simulink model "SF106A_MotRplCoggCfg"  (R2013b)
settings: Solver=FixedStepDiscrete  SolverMode=SingleTasking  StartTime=0.0  StopTime=1  FixedStep=0.002  RelTol=1e-3
undefined symbols (not defined in the file): ARCHGLBPRM_2PI_ULS_F32, ARCHGLBPRM_FLOATZEROTHD_ULS_F32, ARCHGLBPRM_HALFSQRT3_ULS_F32, COGGORDER1_CNT_U16, COGGORDER2_CNT_U16, COGGORDER3_CNT_U16, magnitude, MotCtrlPrmEstimnMotBackEmfConNom, MotRplCoggCfgMotAgTiDly, MotRplCoggCfgMotCurrDaxRplBilnrSeln, MotRplCoggCfgMotCurrQaxRpl, MotRplCoggCfgMotTqRplOrder1X, MotRplCoggCfgMotTqRplOrder1Y, MotRplCoggCfgMotTqRplOrder2X, MotRplCoggCfgMotTqRplOrder2Y, MotRplCoggCfgMotTqRplOrder3X, MotRplCoggCfgMotTqRplOrder3Y, MotRplCoggCmdHrmncOrder1Elec, MotRplCoggCmdHrmncOrder2Elec, MotRplCoggCmdHrmncOrder3Elec, NvmGetErrSts1, ONEOVER2_ULS_F32, SysGlbPrmMotPoleCnt, THREEOVER8_ULS_F32
libraries: NxtrLim x20, FixdToFloat x12, FloatToFixd x6, BilnrIntrpnCmnX x6, BilnrIntrpnCmnXDyn x6, NxtrMath x6, NxtrAbslt x5, NxtrNvM x3, simulink x2, NxtrSign x2
(part 2 of 3)

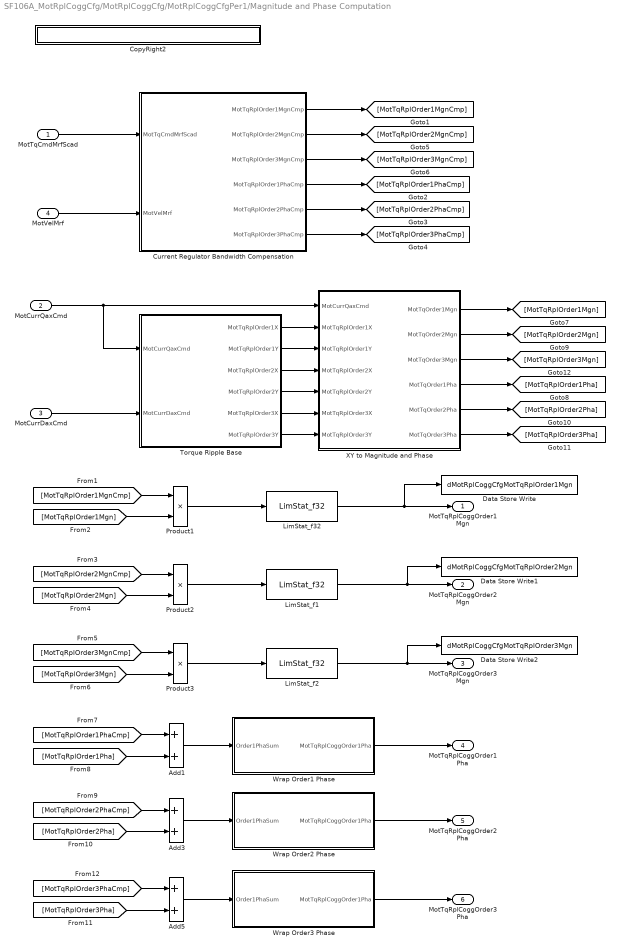
== system SF106A_MotRplCoggCfg/MotRplCoggCfg/MotRplCoggCfgPer1/Magnitude and Phase Computation ==
  MotTqCmdMrfScad : Inport
  MotCurrQaxCmd : Inport  Port=2
  MotCurrDaxCmd : Inport  Port=3
  MotVelMrf : Inport  Port=4
  Add1 : Sum  RequirementInfo="{'linktype_rmi_doors' '0000bb45 (/E-STEER Core/SubSystem Specifications/Application Functions/SF99/SF106A Cogging and Ripple Configuration)' '#SF106A_71' 'true' 'REQ:  SF106A_71' '' } %GIDa_648c56d2_593f_4874_8e89_241910faf26d"
  Add3 : Sum  RequirementInfo="{'linktype_rmi_doors' '0000bb45 (/E-STEER Core/SubSystem Specifications/Application Functions/SF99/SF106A Cogging and Ripple Configuration)' '#SF106A_71' 'true' 'REQ:  SF106A_71' '' } %GIDa_9a9eb539_2504_450c_99aa_20a14d3eef33"
  Add5 : Sum  RequirementInfo="{'linktype_rmi_doors' '0000bb45 (/E-STEER Core/SubSystem Specifications/Application Functions/SF99/SF106A Cogging and Ripple Configuration)' '#SF106A_71' 'true' 'REQ:  SF106A_71' '' } %GIDa_c4a088ef_46a4_443e_8376_4120059d3c17"
  CopyRight2 : Subsystem  Description=|  mask(Copyright Information){none=on}
      | Copyright info block.                                               
      |                                                                     
      | Place copyright information at the top of every subsystem in design.
      mask prompts: none "No parameters"
      mask help: Place copyright information at the top of every subsystem in design.
      mask Display:
      | NxtrConf = 'Nexteer Confidential';
      | 
      | sys = bdroot; %handle for the current model ("system")
      | first = get_param(sys,'Created');
      | if(isempty(first))
      |     first = datestr(now,'yyyy');
      | else
      |     first = first(end-3:end);  %year is last four digits
      | end
      | 
      | last = get_param(sys,'LastModifiedDate');
      | if isempty(last)
      |     last = datestr(now,'yyyy');
      | else
      |     last = last(end-3:end);
      | end
      | 
      | if strcmp(first,last)
      |     fprintf('%s -- Copyright %s Nexteer',NxtrConf,first)
      | else
      |     fprintf('%s -- %s%s- %s Nexteer',NxtrConf,char(169),first,last)
      | end
  Current Regulator Bandwidth Compensation : Subsystem
  Data Store Write : DataStoreWrite  DataStoreName=dMotRplCoggCfgMotTqRplOrder1Mgn
  Data Store Write1 : DataStoreWrite  DataStoreName=dMotRplCoggCfgMotTqRplOrder2Mgn
  Data Store Write2 : DataStoreWrite  DataStoreName=dMotRplCoggCfgMotTqRplOrder3Mgn
  LimStat_f1 : NxtrLim/LimStat_f32  RequirementInfo="{'linktype_rmi_doors' '0000bb45 (/E-STEER Core/SubSystem Specifications/Application Functions/SF99/SF106A Cogging and Ripple Configuration)' '#SF106A_65' 'true' 'REQ:  SF106A_65' '' } %GIDa_ccff9e31_03fc_44e9_a83d_9653ae9d67c5"  LoLim=MOTTQRPLLOLIM_MOTNWTMTR_F32  HiLim=MOTTQRPLHILIM_MOTNWTMTR_F32
      settings: AttributesFormatString=|
      | Low Limit: %<LoLim>
      | High Limit:%<HiLim>
  LimStat_f2 : NxtrLim/LimStat_f32  RequirementInfo="{'linktype_rmi_doors' '0000bb45 (/E-STEER Core/SubSystem Specifications/Application Functions/SF99/SF106A Cogging and Ripple Configuration)' '#SF106A_65' 'true' 'REQ:  SF106A_65' '' } %GIDa_ae5aa3cb_1ae4_4be4_adae_075219de67e5"  LoLim=MOTTQRPLLOLIM_MOTNWTMTR_F32  HiLim=MOTTQRPLHILIM_MOTNWTMTR_F32
      settings: AttributesFormatString=|
      | Low Limit: %<LoLim>
      | High Limit:%<HiLim>
  LimStat_f32 : NxtrLim/LimStat_f32  RequirementInfo="{'linktype_rmi_doors' '0000bb45 (/E-STEER Core/SubSystem Specifications/Application Functions/SF99/SF106A Cogging and Ripple Configuration)' '#SF106A_65' 'true' 'REQ:  SF106A_65' '' } %GIDa_ba4c2155_2466_4bb3_b693_debdd3d2d6c5"  LoLim=MOTTQRPLLOLIM_MOTNWTMTR_F32  HiLim=MOTTQRPLHILIM_MOTNWTMTR_F32
      settings: AttributesFormatString=|
      | Low Limit: %<LoLim>
      | High Limit:%<HiLim>
  Product1 : Product  RequirementInfo="{'linktype_rmi_doors' '0000bb45 (/E-STEER Core/SubSystem Specifications/Application Functions/SF99/SF106A Cogging and Ripple Configuration)' '#SF106A_70' 'true' 'REQ:  SF106A_70' '' } %GIDa_7ac384b6_01f3_4e7b_b1d7_d1b5b6b1e867"
  Product2 : Product  RequirementInfo="{'linktype_rmi_doors' '0000bb45 (/E-STEER Core/SubSystem Specifications/Application Functions/SF99/SF106A Cogging and Ripple Configuration)' '#SF106A_70' 'true' 'REQ:  SF106A_70' '' } %GIDa_9c353b42_6df7_4475_b5bc_a373fdcf9e44"
  Product3 : Product  RequirementInfo="{'linktype_rmi_doors' '0000bb45 (/E-STEER Core/SubSystem Specifications/Application Functions/SF99/SF106A Cogging and Ripple Configuration)' '#SF106A_70' 'true' 'REQ:  SF106A_70' '' } %GIDa_458a2e09_2cf4_40dd_a1d9_b337fe68f59e"
  Torque Ripple Base : Subsystem
  Wrap Order1 Phase : Subsystem  RequirementInfo="{'linktype_rmi_doors' '0000bb45 (/E-STEER Core/SubSystem Specifications/Application Functions/SF99/SF106A Cogging and Ripple Configuration)' '#SF106A_72' 'true' 'REQ:  SF106A_72' '' } %GIDa_d597ade6_de24_47ef_a527_55bbe8aaa597"
  Wrap Order2 Phase : Subsystem  RequirementInfo="{'linktype_rmi_doors' '0000bb45 (/E-STEER Core/SubSystem Specifications/Application Functions/SF99/SF106A Cogging and Ripple Configuration)' '#SF106A_72' 'true' 'REQ:  SF106A_72' '' } %GIDa_7d28c792_5d3e_45ce_b917_447f54703099"
  Wrap Order3 Phase : Subsystem  RequirementInfo="{'linktype_rmi_doors' '0000bb45 (/E-STEER Core/SubSystem Specifications/Application Functions/SF99/SF106A Cogging and Ripple Configuration)' '#SF106A_72' 'true' 'REQ:  SF106A_72' '' } %GIDa_e3528b43_aef0_489e_91c9_b2e9623abd20"
  XY to Magnitude and Phase : Subsystem
  MotTqRplCoggOrder1Mgn : Outport
  MotTqRplCoggOrder2Mgn : Outport  Port=2
  MotTqRplCoggOrder3Mgn : Outport  Port=3
  MotTqRplCoggOrder1Pha : Outport  Port=4
  MotTqRplCoggOrder2Pha : Outport  Port=5
  MotTqRplCoggOrder3Pha : Outport  Port=6
  wires:
  MotTqCmdMrfScad/1 -> Current Regulator Bandwidth Compensation/1(MotTqCmdMrfScad)
  MotCurrDaxCmd/1 -> Torque Ripple Base/2(MotCurrDaxCmd)
  Torque Ripple Base/6(MotTqRplOrder3Y) -> XY to Magnitude and Phase/7(MotTqRplOrder3Y)
  Torque Ripple Base/5(MotTqRplOrder3X) -> XY to Magnitude and Phase/6(MotTqRplOrder3X)
  Torque Ripple Base/1(MotTqRplOrder1X) -> XY to Magnitude and Phase/2(MotTqRplOrder1X)
  Torque Ripple Base/4(MotTqRplOrder2Y) -> XY to Magnitude and Phase/5(MotTqRplOrder2Y)
  Torque Ripple Base/2(MotTqRplOrder1Y) -> XY to Magnitude and Phase/3(MotTqRplOrder1Y)
  Torque Ripple Base/3(MotTqRplOrder2X) -> XY to Magnitude and Phase/4(MotTqRplOrder2X)
  MotCurrQaxCmd/1 -> XY to Magnitude and Phase/1(MotCurrQaxCmd), Torque Ripple Base/1(MotCurrQaxCmd)
  LimStat_f2/1 -> Data Store Write2/1, MotTqRplCoggOrder3Mgn/1
  LimStat_f1/1 -> MotTqRplCoggOrder2Mgn/1, Data Store Write1/1
  LimStat_f32/1 -> MotTqRplCoggOrder1Mgn/1, Data Store Write/1
  MotVelMrf/1 -> Current Regulator Bandwidth Compensation/2(MotVelMrf)
  Product1/1 -> LimStat_f32/1
  [MotTqRplOrder1MgnCmp] -> Product1/1
  [MotTqRplOrder1Mgn] -> Product1/2
  Product2/1 -> LimStat_f1/1
  [MotTqRplOrder2MgnCmp] -> Product2/1
  [MotTqRplOrder2Mgn] -> Product2/2
  Product3/1 -> LimStat_f2/1
  [MotTqRplOrder3MgnCmp] -> Product3/1
  [MotTqRplOrder3Mgn] -> Product3/2
  [MotTqRplOrder1Pha] -> Add1/2
  [MotTqRplOrder1PhaCmp] -> Add1/1
  [MotTqRplOrder2Pha] -> Add3/2
  [MotTqRplOrder2PhaCmp] -> Add3/1
  [MotTqRplOrder3Pha] -> Add5/2
  [MotTqRplOrder3PhaCmp] -> Add5/1
  Add1/1 -> Wrap Order1 Phase/1(Order1PhaSum)
  Wrap Order1 Phase/1(MotTqRplCoggOrder1Pha) -> MotTqRplCoggOrder1Pha/1
  Add3/1 -> Wrap Order2 Phase/1(Order1PhaSum)
  Wrap Order2 Phase/1(MotTqRplCoggOrder1Pha) -> MotTqRplCoggOrder2Pha/1
  Add5/1 -> Wrap Order3 Phase/1(Order1PhaSum)
  Wrap Order3 Phase/1(MotTqRplCoggOrder1Pha) -> MotTqRplCoggOrder3Pha/1
  XY to Magnitude and Phase/1(MotTqOrder1Mgn) -> [MotTqRplOrder1Mgn]
  XY to Magnitude and Phase/3(MotTqOrder3Mgn) -> [MotTqRplOrder3Mgn]
  XY to Magnitude and Phase/5(MotTqOrder2Pha) -> [MotTqRplOrder2Pha]
  XY to Magnitude and Phase/2(MotTqOrder2Mgn) -> [MotTqRplOrder2Mgn]
  XY to Magnitude and Phase/6(MotTqOrder3Pha) -> [MotTqRplOrder3Pha]
  XY to Magnitude and Phase/4(MotTqOrder1Pha) -> [MotTqRplOrder1Pha]
  Current Regulator Bandwidth Compensation/4(MotTqRplOrder1PhaCmp) -> [MotTqRplOrder1PhaCmp]
  Current Regulator Bandwidth Compensation/2(MotTqRplOrder2MgnCmp) -> [MotTqRplOrder2MgnCmp]
  Current Regulator Bandwidth Compensation/3(MotTqRplOrder3MgnCmp) -> [MotTqRplOrder3MgnCmp]
  Current Regulator Bandwidth Compensation/6(MotTqRplOrder3PhaCmp) -> [MotTqRplOrder3PhaCmp]
  Current Regulator Bandwidth Compensation/1(MotTqRplOrder1MgnCmp) -> [MotTqRplOrder1MgnCmp]
  Current Regulator Bandwidth Compensation/5(MotTqRplOrder2PhaCmp) -> [MotTqRplOrder2PhaCmp]

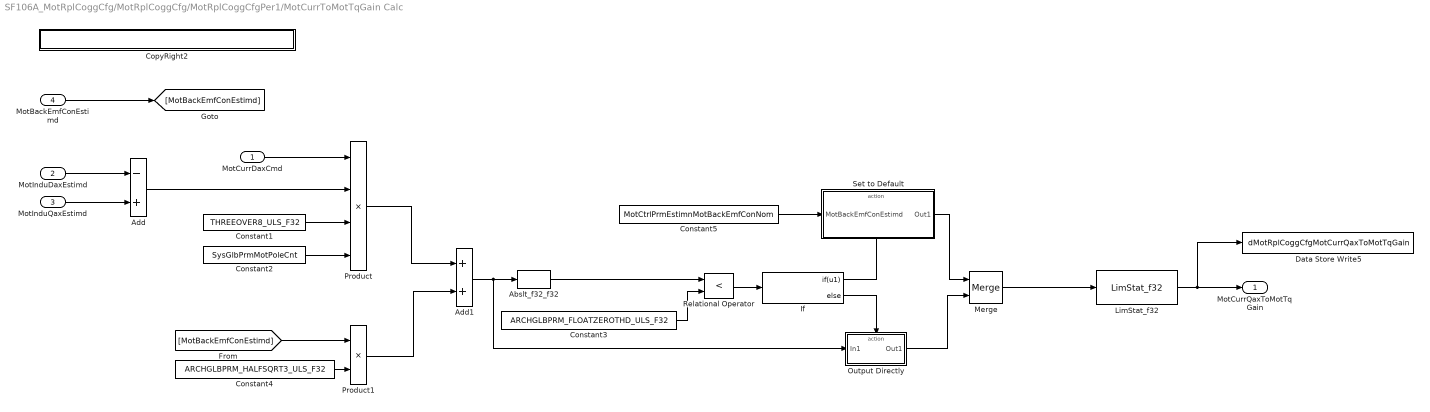
== system SF106A_MotRplCoggCfg/MotRplCoggCfg/MotRplCoggCfgPer1/MotCurrToMotTqGain Calc ==
  MotCurrDaxCmd : Inport
  MotInduDaxEstimd : Inport  Port=2
  MotInduQaxEstimd : Inport  Port=3
  MotBackEmfConEstimd : Inport  Port=4
  Abslt_f32_f32 : NxtrAbslt/Abslt_f32_f32  RequirementInfo="{'linktype_rmi_doors' '0000bb45 (/E-STEER Core/SubSystem Specifications/Application Functions/SF99/SF106A Cogging and Ripple Configuration)' '#SF106A_56' 'true' 'REQ:  SF106A_56' '' } %GIDa_3dd04d32_cbb3_4f3b_a584_375cf79a7190"  SFunctionSpec=single y1 = Abslt_f32_f32(single u1)
      settings: AttributesFormatString=%<Name>
  Add : Sum  RequirementInfo="{'linktype_rmi_doors' '0000bb45 (/E-STEER Core/SubSystem Specifications/Application Functions/SF99/SF106A Cogging and Ripple Configuration)' '#SF106A_54' 'true' 'REQ:  SF106A_54' '' } %GIDa_ba1b20c0_2ede_4be5_979a_b04b55223ef1"  Inputs=-+
  Add1 : Sum  RequirementInfo="{'linktype_rmi_doors' '0000bb45 (/E-STEER Core/SubSystem Specifications/Application Functions/SF99/SF106A Cogging and Ripple Configuration)' '#SF106A_54' 'true' 'REQ:  SF106A_54' '' } %GIDa_ee9a033f_945c_4511_8002_119d863c4908"
  Constant1 : Constant  Value=THREEOVER8_ULS_F32
  Constant2 : Constant  Value=SysGlbPrmMotPoleCnt
  Constant3 : Constant  Value=ARCHGLBPRM_FLOATZEROTHD_ULS_F32
  Constant4 : Constant  Value=ARCHGLBPRM_HALFSQRT3_ULS_F32
  Constant5 : Constant  RequirementInfo={'linktype_rmi_doors' '0000bb45 (/E-STEER Core/SubSystem Specifications/Application Functions/SF99/SF106A Cogging and Ripple Configuration)' '#SF106A_115' 'true' 'REQ: SF106A_115' '' } %GIDa_32d27978_b4ee_4bc2_b947_2a7fafd2bf6c  Value=MotCtrlPrmEstimnMotBackEmfConNom
  CopyRight2 : Subsystem  Description=|  mask(Copyright Information){none=on}
      | Copyright info block.                                               
      |                                                                     
      | Place copyright information at the top of every subsystem in design.
      mask prompts: none "No parameters"
      mask help: Place copyright information at the top of every subsystem in design.
      mask Display:
      | NxtrConf = 'Nexteer Confidential';
      | 
      | sys = bdroot; %handle for the current model ("system")
      | first = get_param(sys,'Created');
      | if(isempty(first))
      |     first = datestr(now,'yyyy');
      | else
      |     first = first(end-3:end);  %year is last four digits
      | end
      | 
      | last = get_param(sys,'LastModifiedDate');
      | if isempty(last)
      |     last = datestr(now,'yyyy');
      | else
      |     last = last(end-3:end);
      | end
      | 
      | if strcmp(first,last)
      |     fprintf('%s -- Copyright %s Nexteer',NxtrConf,first)
      | else
      |     fprintf('%s -- %s%s- %s Nexteer',NxtrConf,char(169),first,last)
      | end
  Data Store Write5 : DataStoreWrite  DataStoreName=dMotRplCoggCfgMotCurrQaxToMotTqGain
  If : If  RequirementInfo="{'linktype_rmi_doors' '0000bb45 (/E-STEER Core/SubSystem Specifications/Application Functions/SF99/SF106A Cogging and Ripple Configuration)' '#SF106A_56' 'true' 'REQ:  SF106A_56' '' ; 'linktype_rmi_doors' '0000bb45 (/E-STEER Core/SubSystem Specifications/Application Functions/SF99/SF106A Cogging and Ripple Configuration)' '#SF106A_56' 'true' 'REQ:  SF106A_56' '' } %GIDa_a5d88a30_9910_4f5f_9fc9_b7b9a6575954"  IfExpression=u1
  LimStat_f32 : NxtrLim/LimStat_f32  LoLim=MOTCURRQAXTOMOTTQGAINLOLIM_VOLTPERMOTRADPERSEC_F32  HiLim=MOTCURRQAXTOMOTTQGAINHILIM_VOLTPERMOTRADPERSEC_F32
      settings: AttributesFormatString=|
      | Low Limit: %<LoLim>
      | High Limit:%<HiLim>
  Merge : Merge  RequirementInfo="{'linktype_rmi_doors' '0000bb45 (/E-STEER Core/SubSystem Specifications/Application Functions/SF99/SF106A Cogging and Ripple Configuration)' '#SF106A_56' 'true' 'REQ:  SF106A_56' '' } %GIDa_c0409470_3f74_4a50_ab79_400dfe325cdd"
  Output Directly : Subsystem  RequirementInfo="{'linktype_rmi_doors' '0000bb45 (/E-STEER Core/SubSystem Specifications/Application Functions/SF99/SF106A Cogging and Ripple Configuration)' '#SF106A_56' 'true' 'REQ:  SF106A_56' '' } %GIDa_2b70c7c7_a78b_446c_bf60_f39fcd5329cf"  TreatAsAtomicUnit=on
  Product : Product  RequirementInfo="{'linktype_rmi_doors' '0000bb45 (/E-STEER Core/SubSystem Specifications/Application Functions/SF99/SF106A Cogging and Ripple Configuration)' '#SF106A_54' 'true' 'REQ:  SF106A_54' '' } %GIDa_d7691117_ecce_48e1_9f0c_630d5d46c3ee"  Inputs=4
  Product1 : Product  RequirementInfo="{'linktype_rmi_doors' '0000bb45 (/E-STEER Core/SubSystem Specifications/Application Functions/SF99/SF106A Cogging and Ripple Configuration)' '#SF106A_54' 'true' 'REQ:  SF106A_54' '' } %GIDa_d73ba26f_a7f2_4740_a78f_0423572b7171"
  Relational Operator : RelationalOperator  RequirementInfo="{'linktype_rmi_doors' '0000bb45 (/E-STEER Core/SubSystem Specifications/Application Functions/SF99/SF106A Cogging and Ripple Configuration)' '#SF106A_56' 'true' 'REQ:  SF106A_56' '' } %GIDa_6b39b974_a2b5_4090_81ce_b211ed84d319"  Operator=<  OutDataTypeStr=boolean
  Set to Default : Subsystem  RequirementInfo="{'linktype_rmi_doors' '0000bb45 (/E-STEER Core/SubSystem Specifications/Application Functions/SF99/SF106A Cogging and Ripple Configuration)' '#SF106A_56' 'true' 'REQ:  SF106A_56' '' } %GIDa_e7fae6b2_5e55_4c14_bb87_5e4affbd739c"  TreatAsAtomicUnit=on
  MotCurrQaxToMotTqGain : Outport
  wires:
  MotInduQaxEstimd/1 -> Add/2
  MotInduDaxEstimd/1 -> Add/1
  Add/1 -> Product/2
  Constant2/1 -> Product/4
  Constant1/1 -> Product/3
  Constant4/1 -> Product1/2
  MotBackEmfConEstimd/1 -> [MotBackEmfConEstimd]
  MotCurrDaxCmd/1 -> Product/1
  Product/1 -> Add1/1
  Product1/1 -> Add1/2
  Add1/1 -> Output Directly/1(In1), Abslt_f32_f32/1
  If/2 -> Output Directly/Action
  If/1 -> Set to Default/Action
  Set to Default/1(Out1) -> Merge/1
  Output Directly/1(Out1) -> Merge/2
  [MotBackEmfConEstimd] -> Product1/1
  Merge/1 -> LimStat_f32/1
  Abslt_f32_f32/1 -> Relational Operator/1
  LimStat_f32/1 -> Data Store Write5/1, MotCurrQaxToMotTqGain/1
  Relational Operator/1 -> If/1
  Constant3/1 -> Relational Operator/2
  Constant5/1 -> Set to Default/1(MotBackEmfConEstimd)

== system SF106A_MotRplCoggCfg/MotRplCoggCfg/MotRplCoggCfgPer1/Position Delay ==
  MotVelMrf : Inport
  Constant : Constant  Value=SysGlbPrmMotPoleCnt
  Constant1 : Constant  Value=ONEOVER2_ULS_F32
  Constant2 : Constant  Value=MotRplCoggCfgMotAgTiDly
  CopyRight2 : Subsystem  Description=|  mask(Copyright Information){none=on}
      | Copyright info block.                                               
      |                                                                     
      | Place copyright information at the top of every subsystem in design.
      mask prompts: none "No parameters"
      mask help: Place copyright information at the top of every subsystem in design.
      mask Display:
      | NxtrConf = 'Nexteer Confidential';
      | 
      | sys = bdroot; %handle for the current model ("system")
      | first = get_param(sys,'Created');
      | if(isempty(first))
      |     first = datestr(now,'yyyy');
      | else
      |     first = first(end-3:end);  %year is last four digits
      | end
      | 
      | last = get_param(sys,'LastModifiedDate');
      | if isempty(last)
      |     last = datestr(now,'yyyy');
      | else
      |     last = last(end-3:end);
      | end
      | 
      | if strcmp(first,last)
      |     fprintf('%s -- Copyright %s Nexteer',NxtrConf,first)
      | else
      |     fprintf('%s -- %s%s- %s Nexteer',NxtrConf,char(169),first,last)
      | end
  Data Store Write5 : DataStoreWrite  DataStoreName=dMotRplCoggCfgMotAgElecDlyRpl
  LimStat_f32 : NxtrLim/LimStat_f32  LoLim=MOTAGELECDLYRPLLOLIM_MOTRAD_F32  HiLim=MOTAGELECDLYRPLHILIM_MOTRAD_F32
      settings: AttributesFormatString=|
      | Low Limit: %<LoLim>
      | High Limit:%<HiLim>
  Product : Product  RequirementInfo="{'linktype_rmi_doors' '0000bb45 (/E-STEER Core/SubSystem Specifications/Application Functions/SF99/SF106A Cogging and Ripple Configuration)' '#SF106A_79' 'true' 'REQ:  SF106A_79' '' } %GIDa_afe57c97_f375_490a_8df4_4de7a5eb3ebb"  Inputs=4
  MotAgElecDlyRpl : Outport
  wires:
  MotVelMrf/1 -> Product/1
  Constant2/1 -> Product/2
  Constant/1 -> Product/3
  Constant1/1 -> Product/4
  Product/1 -> LimStat_f32/1
  LimStat_f32/1 -> Data Store Write5/1, MotAgElecDlyRpl/1

== system SF106A_MotRplCoggCfg/MotRplCoggCfg/SetMotRplCoggPrm/CopyRight2 ==

== system SF106A_MotRplCoggCfg/MotRplCoggCfg/MotRplCoggCfgInit1/NVM is NOT okay/CopyRight2 ==

== system SF106A_MotRplCoggCfg/MotRplCoggCfg/MotRplCoggCfgInit1/NVM is okay/CopyRight2 ==

== system SF106A_MotRplCoggCfg/MotRplCoggCfg/MotRplCoggCfgPer1/Magnitude and Phase Computation/CopyRight2 ==

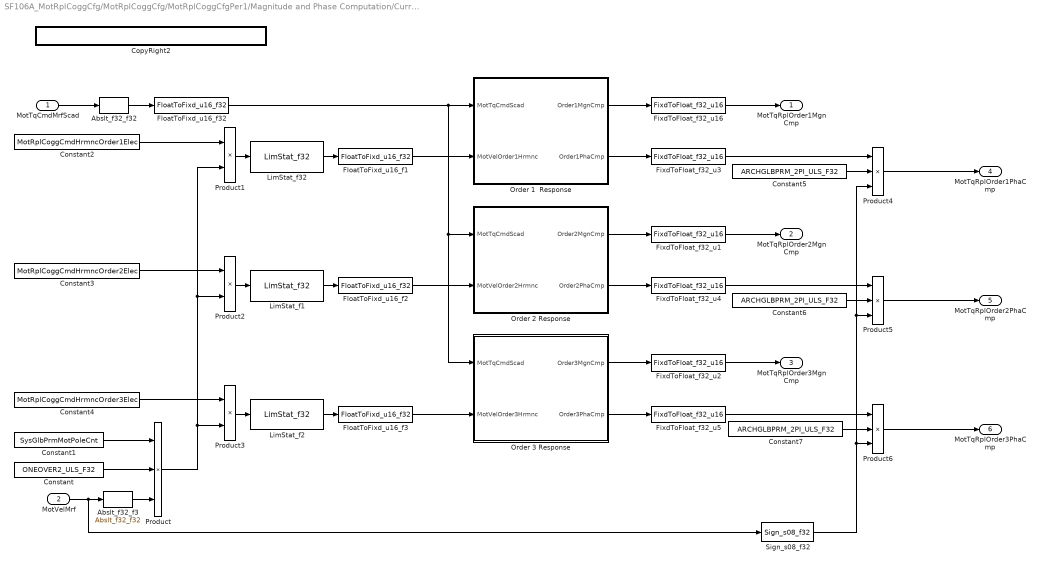
== system SF106A_MotRplCoggCfg/MotRplCoggCfg/MotRplCoggCfgPer1/Magnitude and Phase Computation/Current Regulator Bandwidth Compensation ==
  MotTqCmdMrfScad : Inport
  MotVelMrf : Inport  Port=2
  Abslt_f32_f3 : NxtrAbslt/Abslt_f32_f32  RequirementInfo="{'linktype_rmi_doors' '0000bb45 (/E-STEER Core/SubSystem Specifications/Application Functions/SF99/SF106A Cogging and Ripple Configuration)' '#SF106A_67' 'true' 'REQ:  SF106A_67' '' ; 'linktype_rmi_doors' '0000bb45 (/E-STEER Core/SubSystem Specifications/Application Functions/SF99/SF106A Cogging and Ripple Configuration)' '#SF106A_68' 'true' 'REQ:  SF106A_68' '' } %GIDa_33edf65c_2e46_411e_8167_82b34b9b363e"  SFunctionSpec=single y1 = Abslt_f32_f32(single u1)
      settings: AttributesFormatString=%<Name>
  Abslt_f32_f32 : NxtrAbslt/Abslt_f32_f32  RequirementInfo="{'linktype_rmi_doors' '0000bb45 (/E-STEER Core/SubSystem Specifications/Application Functions/SF99/SF106A Cogging and Ripple Configuration)' '#SF106A_67' 'true' 'REQ:  SF106A_67' '' ; 'linktype_rmi_doors' '0000bb45 (/E-STEER Core/SubSystem Specifications/Application Functions/SF99/SF106A Cogging and Ripple Configuration)' '#SF106A_68' 'true' 'REQ:  SF106A_68' '' } %GIDa_7d0e2c5c_7282_4961_ba80_71904d67d8ed"  SFunctionSpec=single y1 = Abslt_f32_f32(single u1)
      settings: AttributesFormatString=%<Name>
  Constant : Constant  Value=ONEOVER2_ULS_F32
  Constant1 : Constant  Value=SysGlbPrmMotPoleCnt
  Constant2 : Constant  Value=MotRplCoggCmdHrmncOrder1Elec
  Constant3 : Constant  Value=MotRplCoggCmdHrmncOrder2Elec
  Constant4 : Constant  Value=MotRplCoggCmdHrmncOrder3Elec
  Constant5 : Constant  Value=ARCHGLBPRM_2PI_ULS_F32
  Constant6 : Constant  Value=ARCHGLBPRM_2PI_ULS_F32
  Constant7 : Constant  Value=ARCHGLBPRM_2PI_ULS_F32
  CopyRight2 : Subsystem  Description=|  mask(Copyright Information){none=on}
      | Copyright info block.                                               
      |                                                                     
      | Place copyright information at the top of every subsystem in design.
      mask prompts: none "No parameters"
      mask help: Place copyright information at the top of every subsystem in design.
      mask Display:
      | NxtrConf = 'Nexteer Confidential';
      | 
      | sys = bdroot; %handle for the current model ("system")
      | first = get_param(sys,'Created');
      | if(isempty(first))
      |     first = datestr(now,'yyyy');
      | else
      |     first = first(end-3:end);  %year is last four digits
      | end
      | 
      | last = get_param(sys,'LastModifiedDate');
      | if isempty(last)
      |     last = datestr(now,'yyyy');
      | else
      |     last = last(end-3:end);
      | end
      | 
      | if strcmp(first,last)
      |     fprintf('%s -- Copyright %s Nexteer',NxtrConf,first)
      | else
      |     fprintf('%s -- %s%s- %s Nexteer',NxtrConf,char(169),first,last)
      | end
  FixdToFloat_f32_u1 : FixdToFloat/FixdToFloat_f32_u16  Param1=13
  FixdToFloat_f32_u16 : FixdToFloat/FixdToFloat_f32_u16  Param1=13
  FixdToFloat_f32_u2 : FixdToFloat/FixdToFloat_f32_u16  Param1=13
  FixdToFloat_f32_u3 : FixdToFloat/FixdToFloat_f32_u16  Param1=16
  FixdToFloat_f32_u4 : FixdToFloat/FixdToFloat_f32_u16  Param1=16
  FixdToFloat_f32_u5 : FixdToFloat/FixdToFloat_f32_u16  Param1=16
  FloatToFixd_u16_f1 : FloatToFixd/FloatToFixd_u16_f32  Param1=0
  FloatToFixd_u16_f2 : FloatToFixd/FloatToFixd_u16_f32  Param1=0
  FloatToFixd_u16_f3 : FloatToFixd/FloatToFixd_u16_f32  Param1=0
  FloatToFixd_u16_f32 : FloatToFixd/FloatToFixd_u16_f32  Param1=11
  LimStat_f1 : NxtrLim/LimStat_f32  LoLim=SCADMOTVELLOLIM_MOTRADPERSEC_F32  HiLim=SCADMOTVELHILIM_MOTRADPERSEC_F32
      settings: AttributesFormatString=|
      | Low Limit: %<LoLim>
      | High Limit:%<HiLim>
  LimStat_f2 : NxtrLim/LimStat_f32  LoLim=SCADMOTVELLOLIM_MOTRADPERSEC_F32  HiLim=SCADMOTVELHILIM_MOTRADPERSEC_F32
      settings: AttributesFormatString=|
      | Low Limit: %<LoLim>
      | High Limit:%<HiLim>
  LimStat_f32 : NxtrLim/LimStat_f32  LoLim=SCADMOTVELLOLIM_MOTRADPERSEC_F32  HiLim=SCADMOTVELHILIM_MOTRADPERSEC_F32
      settings: AttributesFormatString=|
      | Low Limit: %<LoLim>
      | High Limit:%<HiLim>
  Order 1  Response : Subsystem
  Order 2 Response : Subsystem
  Order 3 Response : Subsystem
  Product : Product  RequirementInfo="{'linktype_rmi_doors' '0000bb45 (/E-STEER Core/SubSystem Specifications/Application Functions/SF99/SF106A Cogging and Ripple Configuration)' '#SF106A_81' 'true' 'REQ:  SF106A_81' '' } %GIDa_c32ba144_8f46_4563_9287_d3fbee22e8ee"  Inputs=3
  Product1 : Product  RequirementInfo="{'linktype_rmi_doors' '0000bb45 (/E-STEER Core/SubSystem Specifications/Application Functions/SF99/SF106A Cogging and Ripple Configuration)' '#SF106A_81' 'true' 'REQ:  SF106A_81' '' } %GIDa_53901d07_6f3a_4129_bea4_9e1cfca6b240"
  Product2 : Product  RequirementInfo="{'linktype_rmi_doors' '0000bb45 (/E-STEER Core/SubSystem Specifications/Application Functions/SF99/SF106A Cogging and Ripple Configuration)' '#SF106A_81' 'true' 'REQ:  SF106A_81' '' } %GIDa_502d1333_b67d_4aee_b399_61be2d4ee1b7"
  Product3 : Product  RequirementInfo="{'linktype_rmi_doors' '0000bb45 (/E-STEER Core/SubSystem Specifications/Application Functions/SF99/SF106A Cogging and Ripple Configuration)' '#SF106A_81' 'true' 'REQ:  SF106A_81' '' } %GIDa_398cdf39_2b12_4b5d_a0f8_77f90bad82f0"
  Product4 : Product  Inputs=3
  Product5 : Product  Inputs=3
  Product6 : Product  Inputs=3
  Sign_s08_f32 : NxtrSign/Sign_s08_f32  SFunctionSpec=int8 y1 = Sign_s08_f32(single u1)
  MotTqRplOrder1MgnCmp : Outport
  MotTqRplOrder2MgnCmp : Outport  Port=2
  MotTqRplOrder3MgnCmp : Outport  Port=3
  MotTqRplOrder1PhaCmp : Outport  Port=4
  MotTqRplOrder2PhaCmp : Outport  Port=5
  MotTqRplOrder3PhaCmp : Outport  Port=6
  wires:
  MotVelMrf/1 -> Sign_s08_f32/1, Abslt_f32_f3/1
  Constant/1 -> Product/2
  Constant1/1 -> Product/1
  MotTqCmdMrfScad/1 -> Abslt_f32_f32/1
  Abslt_f32_f32/1 -> FloatToFixd_u16_f32/1
  Constant2/1 -> Product1/1
  Product1/1 -> LimStat_f32/1
  Constant3/1 -> Product2/1
  Constant4/1 -> Product3/1
  Product2/1 -> LimStat_f1/1
  Product3/1 -> LimStat_f2/1
  FloatToFixd_u16_f2/1 -> Order 2 Response/2(MotVelOrder2Hrmnc)
  FloatToFixd_u16_f32/1 -> Order 2 Response/1(MotTqCmdScad), Order 3 Response/1(MotTqCmdScad), Order 1  Response/1(MotTqCmdScad)
  FloatToFixd_u16_f1/1 -> Order 1  Response/2(MotVelOrder1Hrmnc)
  Order 1  Response/1(Order1MgnCmp) -> FixdToFloat_f32_u16/1
  Order 1  Response/2(Order1PhaCmp) -> FixdToFloat_f32_u3/1
  FloatToFixd_u16_f3/1 -> Order 3 Response/2(MotVelOrder3Hrmnc)
  FixdToFloat_f32_u16/1 -> MotTqRplOrder1MgnCmp/1
  Constant5/1 -> Product4/2
  Product/1 -> Product3/2, Product1/2, Product2/2
  FixdToFloat_f32_u1/1 -> MotTqRplOrder2MgnCmp/1
  Order 2 Response/1(Order2MgnCmp) -> FixdToFloat_f32_u1/1
  FixdToFloat_f32_u2/1 -> MotTqRplOrder3MgnCmp/1
  Order 3 Response/1(Order3MgnCmp) -> FixdToFloat_f32_u2/1
  Constant6/1 -> Product5/2
  Order 2 Response/2(Order2PhaCmp) -> FixdToFloat_f32_u4/1
  Order 3 Response/2(Order3PhaCmp) -> FixdToFloat_f32_u5/1
  Constant7/1 -> Product6/2
  Sign_s08_f32/1 -> Product6/3, Product5/3, Product4/3
  Product5/1 -> MotTqRplOrder2PhaCmp/1
  Product4/1 -> MotTqRplOrder1PhaCmp/1
  Product6/1 -> MotTqRplOrder3PhaCmp/1
  FixdToFloat_f32_u3/1 -> Product4/1
  FixdToFloat_f32_u4/1 -> Product5/1
  FixdToFloat_f32_u5/1 -> Product6/1
  Abslt_f32_f3/1 -> Product/3
  LimStat_f32/1 -> FloatToFixd_u16_f1/1
  LimStat_f1/1 -> FloatToFixd_u16_f2/1
  LimStat_f2/1 -> FloatToFixd_u16_f3/1

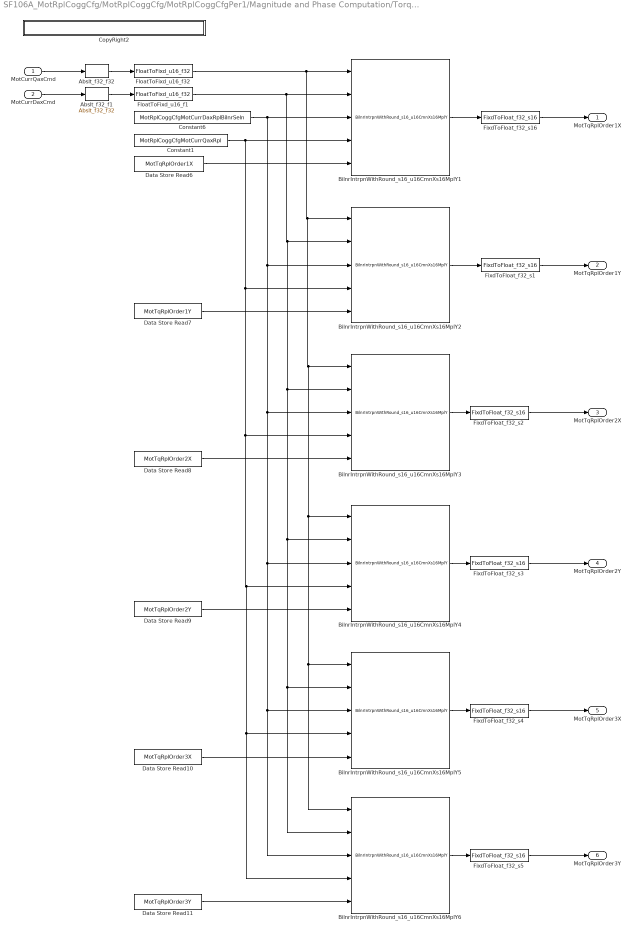
== system SF106A_MotRplCoggCfg/MotRplCoggCfg/MotRplCoggCfgPer1/Magnitude and Phase Computation/Torque Ripple Base ==
  MotCurrQaxCmd : Inport
  MotCurrDaxCmd : Inport  Port=2
  Abslt_f32_f1 : NxtrAbslt/Abslt_f32_f32  RequirementInfo="{'linktype_rmi_doors' '0000bb45 (/E-STEER Core/SubSystem Specifications/Application Functions/SF99/SF106A Cogging and Ripple Configuration)' '#SF106A_60' 'true' 'REQ:  SF106A_60' '' } %GIDa_f23e7e06_4942_429e_aaa7_15d7333418e2"  SFunctionSpec=single y1 = Abslt_f32_f32(single u1)
      settings: AttributesFormatString=%<Name>
  Abslt_f32_f32 : NxtrAbslt/Abslt_f32_f32  RequirementInfo="{'linktype_rmi_doors' '0000bb45 (/E-STEER Core/SubSystem Specifications/Application Functions/SF99/SF106A Cogging and Ripple Configuration)' '#SF106A_60' 'true' 'REQ:  SF106A_60' '' } %GIDa_3387224d_78f6_416f_98c0_914edf0753b3"  SFunctionSpec=single y1 = Abslt_f32_f32(single u1)
      settings: AttributesFormatString=%<Name>
  BilnrIntrpnWithRound_s16_u16CmnXs16MplY1 : BilnrIntrpnCmnXDyn/BilnrIntrpnWithRound_s16_u16CmnXs16MplY  RequirementInfo="{'linktype_rmi_doors' '0000bb45 (/E-STEER Core/SubSystem Specifications/Application Functions/SF99/SF106A Cogging and Ripple Configuration)' '#SF106A_59' 'true' 'REQ:  SF106A_59' '' ; 'linktype_rmi_doors' '0000bb45 (/E-STEER Core/SubSystem Specifications/Application Functions/SF99/SF106A Cogging and Ripple Configuration)' '#SF106A_60' 'true' 'REQ:  SF106A_60' '' } %GIDa_4e40eb88_09c7_4e9a_934d_ce90ff574238"
      settings: AttributesFormatString=Bilnr ( u16CmnX , s16MplY )
  BilnrIntrpnWithRound_s16_u16CmnXs16MplY2 : BilnrIntrpnCmnXDyn/BilnrIntrpnWithRound_s16_u16CmnXs16MplY  RequirementInfo="{'linktype_rmi_doors' '0000bb45 (/E-STEER Core/SubSystem Specifications/Application Functions/SF99/SF106A Cogging and Ripple Configuration)' '#SF106A_59' 'true' 'REQ:  SF106A_59' '' ; 'linktype_rmi_doors' '0000bb45 (/E-STEER Core/SubSystem Specifications/Application Functions/SF99/SF106A Cogging and Ripple Configuration)' '#SF106A_60' 'true' 'REQ:  SF106A_60' '' } %GIDa_9113e5b3_626f_4f22_b26b_1255a04298c4"
      settings: AttributesFormatString=Bilnr ( u16CmnX , s16MplY )
  BilnrIntrpnWithRound_s16_u16CmnXs16MplY3 : BilnrIntrpnCmnXDyn/BilnrIntrpnWithRound_s16_u16CmnXs16MplY  RequirementInfo="{'linktype_rmi_doors' '0000bb45 (/E-STEER Core/SubSystem Specifications/Application Functions/SF99/SF106A Cogging and Ripple Configuration)' '#SF106A_59' 'true' 'REQ:  SF106A_59' '' ; 'linktype_rmi_doors' '0000bb45 (/E-STEER Core/SubSystem Specifications/Application Functions/SF99/SF106A Cogging and Ripple Configuration)' '#SF106A_60' 'true' 'REQ:  SF106A_60' '' } %GIDa_08f27982_c405_4de1_a76e_4c506c7c0983"
      settings: AttributesFormatString=Bilnr ( u16CmnX , s16MplY )
  BilnrIntrpnWithRound_s16_u16CmnXs16MplY4 : BilnrIntrpnCmnXDyn/BilnrIntrpnWithRound_s16_u16CmnXs16MplY  RequirementInfo="{'linktype_rmi_doors' '0000bb45 (/E-STEER Core/SubSystem Specifications/Application Functions/SF99/SF106A Cogging and Ripple Configuration)' '#SF106A_59' 'true' 'REQ:  SF106A_59' '' ; 'linktype_rmi_doors' '0000bb45 (/E-STEER Core/SubSystem Specifications/Application Functions/SF99/SF106A Cogging and Ripple Configuration)' '#SF106A_60' 'true' 'REQ:  SF106A_60' '' } %GIDa_a07b69b4_ab66_45a3_85a3_5ab181b678dc"
      settings: AttributesFormatString=Bilnr ( u16CmnX , s16MplY )
  BilnrIntrpnWithRound_s16_u16CmnXs16MplY5 : BilnrIntrpnCmnXDyn/BilnrIntrpnWithRound_s16_u16CmnXs16MplY  RequirementInfo="{'linktype_rmi_doors' '0000bb45 (/E-STEER Core/SubSystem Specifications/Application Functions/SF99/SF106A Cogging and Ripple Configuration)' '#SF106A_59' 'true' 'REQ:  SF106A_59' '' ; 'linktype_rmi_doors' '0000bb45 (/E-STEER Core/SubSystem Specifications/Application Functions/SF99/SF106A Cogging and Ripple Configuration)' '#SF106A_60' 'true' 'REQ:  SF106A_60' '' } %GIDa_daa1d23a_c372_459d_8cec_c0b05fa3e923"
      settings: AttributesFormatString=Bilnr ( u16CmnX , s16MplY )
  BilnrIntrpnWithRound_s16_u16CmnXs16MplY6 : BilnrIntrpnCmnXDyn/BilnrIntrpnWithRound_s16_u16CmnXs16MplY  RequirementInfo="{'linktype_rmi_doors' '0000bb45 (/E-STEER Core/SubSystem Specifications/Application Functions/SF99/SF106A Cogging and Ripple Configuration)' '#SF106A_59' 'true' 'REQ:  SF106A_59' '' ; 'linktype_rmi_doors' '0000bb45 (/E-STEER Core/SubSystem Specifications/Application Functions/SF99/SF106A Cogging and Ripple Configuration)' '#SF106A_60' 'true' 'REQ:  SF106A_60' '' } %GIDa_2798d0eb_c05a_4c0c_9de5_f8165b407397"
      settings: AttributesFormatString=Bilnr ( u16CmnX , s16MplY )
  Constant1 : Constant  Value=MotRplCoggCfgMotCurrQaxRpl
  Constant6 : Constant  Value=MotRplCoggCfgMotCurrDaxRplBilnrSeln
  CopyRight2 : Subsystem  Description=|  mask(Copyright Information){none=on}
      | Copyright info block.                                               
      |                                                                     
      | Place copyright information at the top of every subsystem in design.
      mask prompts: none "No parameters"
      mask help: Place copyright information at the top of every subsystem in design.
      mask Display:
      | NxtrConf = 'Nexteer Confidential';
      | 
      | sys = bdroot; %handle for the current model ("system")
      | first = get_param(sys,'Created');
      | if(isempty(first))
      |     first = datestr(now,'yyyy');
      | else
      |     first = first(end-3:end);  %year is last four digits
      | end
      | 
      | last = get_param(sys,'LastModifiedDate');
      | if isempty(last)
      |     last = datestr(now,'yyyy');
      | else
      |     last = last(end-3:end);
      | end
      | 
      | if strcmp(first,last)
      |     fprintf('%s -- Copyright %s Nexteer',NxtrConf,first)
      | else
      |     fprintf('%s -- %s%s- %s Nexteer',NxtrConf,char(169),first,last)
      | end
  Data Store Read10 : DataStoreRead  DataStoreName=MotTqRplOrder3X
  Data Store Read11 : DataStoreRead  DataStoreName=MotTqRplOrder3Y
  Data Store Read6 : DataStoreRead  DataStoreName=MotTqRplOrder1X
  Data Store Read7 : DataStoreRead  DataStoreName=MotTqRplOrder1Y
  Data Store Read8 : DataStoreRead  DataStoreName=MotTqRplOrder2X
  Data Store Read9 : DataStoreRead  DataStoreName=MotTqRplOrder2Y
  FixdToFloat_f32_s{1..5,16} (6 alike) : FixdToFloat/FixdToFloat_f32_s16  Param1=14
  FloatToFixd_u16_f1 : FloatToFixd/FloatToFixd_u16_f32  Param1=7
  FloatToFixd_u16_f32 : FloatToFixd/FloatToFixd_u16_f32  Param1=7
  MotTqRplOrder1X : Outport
  MotTqRplOrder1Y : Outport  Port=2
  MotTqRplOrder2X : Outport  Port=3
  MotTqRplOrder2Y : Outport  Port=4
  MotTqRplOrder3X : Outport  Port=5
  MotTqRplOrder3Y : Outport  Port=6
  wires:
  MotCurrQaxCmd/1 -> Abslt_f32_f32/1
  Abslt_f32_f32/1 -> FloatToFixd_u16_f32/1
  Abslt_f32_f1/1 -> FloatToFixd_u16_f1/1
  MotCurrDaxCmd/1 -> Abslt_f32_f1/1
  FloatToFixd_u16_f32/1 -> BilnrIntrpnWithRound_s16_u16CmnXs16MplY1/1, BilnrIntrpnWithRound_s16_u16CmnXs16MplY2/1, BilnrIntrpnWithRound_s16_u16CmnXs16MplY3/1, BilnrIntrpnWithRound_s16_u16CmnXs16MplY4/1, BilnrIntrpnWithRound_s16_u16CmnXs16MplY6/1, BilnrIntrpnWithRound_s16_u16CmnXs16MplY5/1
  Constant6/1 -> BilnrIntrpnWithRound_s16_u16CmnXs16MplY1/3, BilnrIntrpnWithRound_s16_u16CmnXs16MplY2/3, BilnrIntrpnWithRound_s16_u16CmnXs16MplY3/3, BilnrIntrpnWithRound_s16_u16CmnXs16MplY4/3, BilnrIntrpnWithRound_s16_u16CmnXs16MplY6/3, BilnrIntrpnWithRound_s16_u16CmnXs16MplY5/3
  Constant1/1 -> BilnrIntrpnWithRound_s16_u16CmnXs16MplY1/4, BilnrIntrpnWithRound_s16_u16CmnXs16MplY2/4, BilnrIntrpnWithRound_s16_u16CmnXs16MplY3/4, BilnrIntrpnWithRound_s16_u16CmnXs16MplY4/4, BilnrIntrpnWithRound_s16_u16CmnXs16MplY6/4, BilnrIntrpnWithRound_s16_u16CmnXs16MplY5/4
  Data Store Read6/1 -> BilnrIntrpnWithRound_s16_u16CmnXs16MplY1/5
  Data Store Read7/1 -> BilnrIntrpnWithRound_s16_u16CmnXs16MplY2/5
  FloatToFixd_u16_f1/1 -> BilnrIntrpnWithRound_s16_u16CmnXs16MplY1/2, BilnrIntrpnWithRound_s16_u16CmnXs16MplY2/2, BilnrIntrpnWithRound_s16_u16CmnXs16MplY3/2, BilnrIntrpnWithRound_s16_u16CmnXs16MplY4/2, BilnrIntrpnWithRound_s16_u16CmnXs16MplY6/2, BilnrIntrpnWithRound_s16_u16CmnXs16MplY5/2
  Data Store Read8/1 -> BilnrIntrpnWithRound_s16_u16CmnXs16MplY3/5
  Data Store Read9/1 -> BilnrIntrpnWithRound_s16_u16CmnXs16MplY4/5
  Data Store Read10/1 -> BilnrIntrpnWithRound_s16_u16CmnXs16MplY5/5
  Data Store Read11/1 -> BilnrIntrpnWithRound_s16_u16CmnXs16MplY6/5
  BilnrIntrpnWithRound_s16_u16CmnXs16MplY1/1 -> FixdToFloat_f32_s16/1
  BilnrIntrpnWithRound_s16_u16CmnXs16MplY2/1 -> FixdToFloat_f32_s1/1
  BilnrIntrpnWithRound_s16_u16CmnXs16MplY3/1 -> FixdToFloat_f32_s2/1
  BilnrIntrpnWithRound_s16_u16CmnXs16MplY4/1 -> FixdToFloat_f32_s3/1
  BilnrIntrpnWithRound_s16_u16CmnXs16MplY5/1 -> FixdToFloat_f32_s4/1
  BilnrIntrpnWithRound_s16_u16CmnXs16MplY6/1 -> FixdToFloat_f32_s5/1
  FixdToFloat_f32_s16/1 -> MotTqRplOrder1X/1
  FixdToFloat_f32_s1/1 -> MotTqRplOrder1Y/1
  FixdToFloat_f32_s2/1 -> MotTqRplOrder2X/1
  FixdToFloat_f32_s3/1 -> MotTqRplOrder2Y/1
  FixdToFloat_f32_s4/1 -> MotTqRplOrder3X/1
  FixdToFloat_f32_s5/1 -> MotTqRplOrder3Y/1

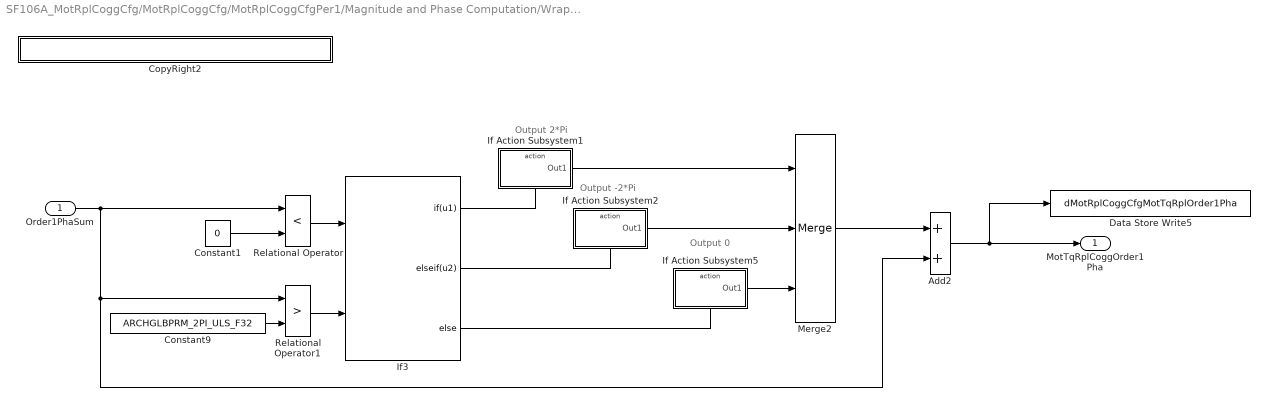
== system SF106A_MotRplCoggCfg/MotRplCoggCfg/MotRplCoggCfgPer1/Magnitude and Phase Computation/Wrap Order1 Phase ==
  note: Output 0
  note: Output 2*Pi
  note: Output -2*Pi
  Order1PhaSum : Inport
  Add2 : Sum
  Constant1 : Constant  Value=0  OutDataTypeStr=single
      settings: AttributesFormatString=%<OutDataTypeStr>
  Constant9 : Constant  Value=ARCHGLBPRM_2PI_ULS_F32
  CopyRight2 : Subsystem  Description=|  mask(Copyright Information){none=on}
      | Copyright info block.                                               
      |                                                                     
      | Place copyright information at the top of every subsystem in design.
      mask prompts: none "No parameters"
      mask help: Place copyright information at the top of every subsystem in design.
      mask Display:
      | NxtrConf = 'Nexteer Confidential';
      | 
      | sys = bdroot; %handle for the current model ("system")
      | first = get_param(sys,'Created');
      | if(isempty(first))
      |     first = datestr(now,'yyyy');
      | else
      |     first = first(end-3:end);  %year is last four digits
      | end
      | 
      | last = get_param(sys,'LastModifiedDate');
      | if isempty(last)
      |     last = datestr(now,'yyyy');
      | else
      |     last = last(end-3:end);
      | end
      | 
      | if strcmp(first,last)
      |     fprintf('%s -- Copyright %s Nexteer',NxtrConf,first)
      | else
      |     fprintf('%s -- %s%s- %s Nexteer',NxtrConf,char(169),first,last)
      | end
  Data Store Write5 : DataStoreWrite  DataStoreName=dMotRplCoggCfgMotTqRplOrder1Pha
  If Action Subsystem1 : Subsystem  TreatAsAtomicUnit=on
  If Action Subsystem2 : Subsystem  TreatAsAtomicUnit=on
  If Action Subsystem5 : Subsystem  TreatAsAtomicUnit=on
  If3 : If  NumInputs=2  IfExpression=u1  ElseIfExpressions=u2
  Merge2 : Merge  Inputs=3
  Relational Operator : RelationalOperator  Operator=<  OutDataTypeStr=boolean
  Relational Operator1 : RelationalOperator  Operator=>  OutDataTypeStr=boolean
  MotTqRplCoggOrder1Pha : Outport
  wires:
  Add2/1 -> MotTqRplCoggOrder1Pha/1, Data Store Write5/1
  If3/3 -> If Action Subsystem5/Action
  If Action Subsystem1/1(Out1) -> Merge2/1
  If Action Subsystem5/1(Out1) -> Merge2/3
  Relational Operator/1 -> If3/1
  Order1PhaSum/1 -> Add2/2, Relational Operator1/1, Relational Operator/1
  Constant1/1 -> Relational Operator/2
  Merge2/1 -> Add2/1
  If3/1 -> If Action Subsystem1/Action
  Constant9/1 -> Relational Operator1/2
  Relational Operator1/1 -> If3/2
  If3/2 -> If Action Subsystem2/Action
  If Action Subsystem2/1(Out1) -> Merge2/2

== system SF106A_MotRplCoggCfg/MotRplCoggCfg/MotRplCoggCfgPer1/Magnitude and Phase Computation/Wrap Order2 Phase ==
  note: Output -2*Pi
  note: Output 2*Pi
  note: Output 0
  Order1PhaSum : Inport
  Add2 : Sum
  Constant1 : Constant  Value=0  OutDataTypeStr=single
      settings: AttributesFormatString=%<OutDataTypeStr>
  Constant9 : Constant  Value=ARCHGLBPRM_2PI_ULS_F32
  CopyRight2 : Subsystem  Description=|  mask(Copyright Information){none=on}
      | Copyright info block.                                               
      |                                                                     
      | Place copyright information at the top of every subsystem in design.
      mask prompts: none "No parameters"
      mask help: Place copyright information at the top of every subsystem in design.
      mask Display:
      | NxtrConf = 'Nexteer Confidential';
      | 
      | sys = bdroot; %handle for the current model ("system")
      | first = get_param(sys,'Created');
      | if(isempty(first))
      |     first = datestr(now,'yyyy');
      | else
      |     first = first(end-3:end);  %year is last four digits
      | end
      | 
      | last = get_param(sys,'LastModifiedDate');
      | if isempty(last)
      |     last = datestr(now,'yyyy');
      | else
      |     last = last(end-3:end);
      | end
      | 
      | if strcmp(first,last)
      |     fprintf('%s -- Copyright %s Nexteer',NxtrConf,first)
      | else
      |     fprintf('%s -- %s%s- %s Nexteer',NxtrConf,char(169),first,last)
      | end
  Data Store Write5 : DataStoreWrite  DataStoreName=dMotRplCoggCfgMotTqRplOrder1Pha
  If Action Subsystem1 : Subsystem  TreatAsAtomicUnit=on
  If Action Subsystem2 : Subsystem  TreatAsAtomicUnit=on
  If Action Subsystem5 : Subsystem  TreatAsAtomicUnit=on
  If3 : If  NumInputs=2  IfExpression=u1  ElseIfExpressions=u2
  Merge2 : Merge  Inputs=3
  Relational Operator : RelationalOperator  Operator=<  OutDataTypeStr=boolean
  Relational Operator1 : RelationalOperator  Operator=>  OutDataTypeStr=boolean
  MotTqRplCoggOrder1Pha : Outport
  wires:
  If Action Subsystem2/1(Out1) -> Merge2/2
  If3/2 -> If Action Subsystem2/Action
  Relational Operator1/1 -> If3/2
  Constant9/1 -> Relational Operator1/2
  If3/1 -> If Action Subsystem1/Action
  Merge2/1 -> Add2/1
  Constant1/1 -> Relational Operator/2
  Order1PhaSum/1 -> Relational Operator/1, Relational Operator1/1, Add2/2
  Relational Operator/1 -> If3/1
  If Action Subsystem5/1(Out1) -> Merge2/3
  If Action Subsystem1/1(Out1) -> Merge2/1
  If3/3 -> If Action Subsystem5/Action
  Add2/1 -> Data Store Write5/1, MotTqRplCoggOrder1Pha/1

== system SF106A_MotRplCoggCfg/MotRplCoggCfg/MotRplCoggCfgPer1/Magnitude and Phase Computation/Wrap Order3 Phase ==
  note: Output 0
  note: Output 2*Pi
  note: Output -2*Pi
  Order1PhaSum : Inport
  Add2 : Sum
  Constant1 : Constant  Value=0  OutDataTypeStr=single
      settings: AttributesFormatString=%<OutDataTypeStr>
  Constant9 : Constant  Value=ARCHGLBPRM_2PI_ULS_F32
  CopyRight2 : Subsystem  Description=|  mask(Copyright Information){none=on}
      | Copyright info block.                                               
      |                                                                     
      | Place copyright information at the top of every subsystem in design.
      mask prompts: none "No parameters"
      mask help: Place copyright information at the top of every subsystem in design.
      mask Display:
      | NxtrConf = 'Nexteer Confidential';
      | 
      | sys = bdroot; %handle for the current model ("system")
      | first = get_param(sys,'Created');
      | if(isempty(first))
      |     first = datestr(now,'yyyy');
      | else
      |     first = first(end-3:end);  %year is last four digits
      | end
      | 
      | last = get_param(sys,'LastModifiedDate');
      | if isempty(last)
      |     last = datestr(now,'yyyy');
      | else
      |     last = last(end-3:end);
      | end
      | 
      | if strcmp(first,last)
      |     fprintf('%s -- Copyright %s Nexteer',NxtrConf,first)
      | else
      |     fprintf('%s -- %s%s- %s Nexteer',NxtrConf,char(169),first,last)
      | end
  Data Store Write5 : DataStoreWrite  DataStoreName=dMotRplCoggCfgMotTqRplOrder1Pha
  If Action Subsystem1 : Subsystem  TreatAsAtomicUnit=on
  If Action Subsystem2 : Subsystem  TreatAsAtomicUnit=on
  If Action Subsystem5 : Subsystem  TreatAsAtomicUnit=on
  If3 : If  NumInputs=2  IfExpression=u1  ElseIfExpressions=u2
  Merge2 : Merge  Inputs=3
  Relational Operator : RelationalOperator  Operator=<  OutDataTypeStr=boolean
  Relational Operator1 : RelationalOperator  Operator=>  OutDataTypeStr=boolean
  MotTqRplCoggOrder1Pha : Outport
  wires:
  Add2/1 -> MotTqRplCoggOrder1Pha/1, Data Store Write5/1
  If3/3 -> If Action Subsystem5/Action
  If Action Subsystem1/1(Out1) -> Merge2/1
  If Action Subsystem5/1(Out1) -> Merge2/3
  Relational Operator/1 -> If3/1
  Order1PhaSum/1 -> Add2/2, Relational Operator1/1, Relational Operator/1
  Constant1/1 -> Relational Operator/2
  Merge2/1 -> Add2/1
  If3/1 -> If Action Subsystem1/Action
  Constant9/1 -> Relational Operator1/2
  Relational Operator1/1 -> If3/2
  If3/2 -> If Action Subsystem2/Action
  If Action Subsystem2/1(Out1) -> Merge2/2
